simulink model "trying_HPF"  (R2024b)
settings: Solver=VariableStepAuto  StartTime=0.0  StopTime=10.0  RelTol=1e-3
libraries: simulink x4, commanapbnd3 x1
settings Model: LastModifiedBy=LENOVO

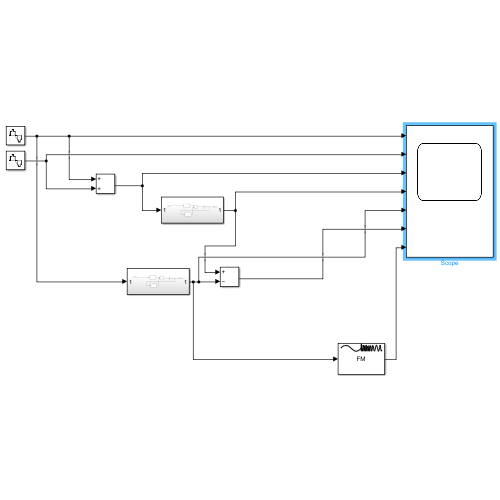
[thumbnail: Simulink's stored preview of the top-level diagram]
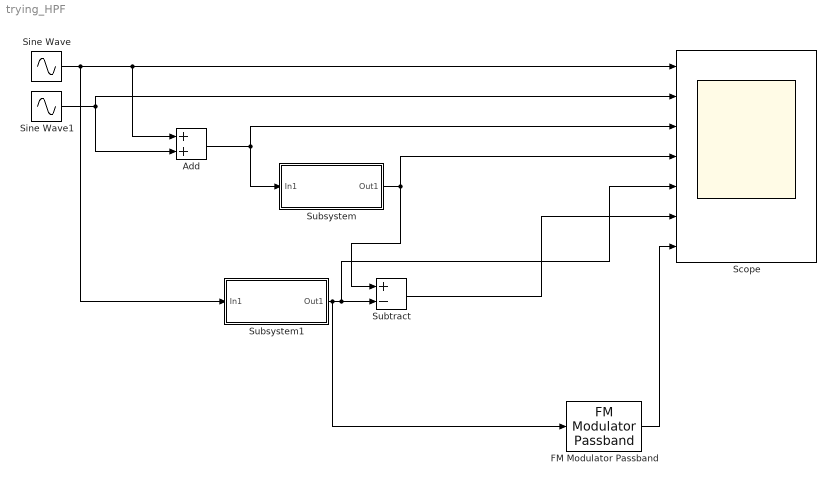
== system trying_HPF ==
  Add : Sum
  FM Modulator Passband : commanapbnd3/FM Modulator Passband  Fc=300  Ph=0  Kc=50
  Scope : Scope  NumInputPorts=7
  Sine Wave : Sin  Amplitude=2  Frequency=2*pi*0.1  SampleTime=0.001
  Sine Wave1 : Sin  Amplitude=2  Frequency=2*pi*2  SampleTime=0.001
  Subsystem : Subsystem
  Subsystem1 : Subsystem
  Subtract : Sum  Inputs=+-
  wires:
  Sine Wave/1 -> Subsystem1/1(In1), Add/1, Scope/1
  Sine Wave1/1 -> Add/2, Scope/2
  Add/1 -> Subsystem/1(In1), Scope/3
  Subsystem/1(Out1) -> Subtract/1, Scope/4
  Subsystem1/1(Out1) -> FM Modulator Passband/1, Scope/5, Subtract/2
  Subtract/1 -> Scope/6
  FM Modulator Passband/1 -> Scope/7

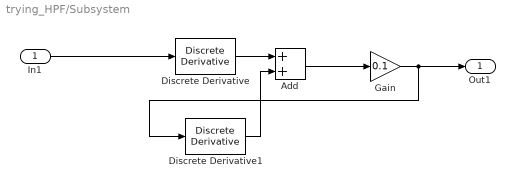
== system trying_HPF/Subsystem ==
  In1 : Inport
  Add : Sum
  Discrete Derivative : simulink/Discrete/Discrete Derivative  gainval=1.0  ICPrevScaledInput=0.0  OutMin=[]  OutMax=[]  OutDataType=fixdt(1, 16)  OutScaling=2^-10  DoSatur=off
  Discrete Derivative1 : simulink/Discrete/Discrete Derivative  gainval=1.0  ICPrevScaledInput=0.0  OutMin=[]  OutMax=[]  OutDataType=fixdt(1, 16)  OutScaling=2^-10  DoSatur=off
  Gain : Gain  Gain=0.1
  Out1 : Outport
  wires:
  Gain/1 -> Discrete Derivative1/1, Out1/1
  Add/1 -> Gain/1
  Discrete Derivative/1 -> Add/1
  In1/1 -> Discrete Derivative/1
  Discrete Derivative1/1 -> Add/2

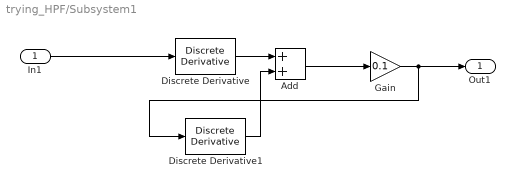
== system trying_HPF/Subsystem1 ==
  In1 : Inport
  Add : Sum
  Discrete Derivative : simulink/Discrete/Discrete Derivative  gainval=1.0  ICPrevScaledInput=0.0  OutMin=[]  OutMax=[]  OutDataType=fixdt(1, 16)  OutScaling=2^-10  DoSatur=off
  Discrete Derivative1 : simulink/Discrete/Discrete Derivative  gainval=1.0  ICPrevScaledInput=0.0  OutMin=[]  OutMax=[]  OutDataType=fixdt(1, 16)  OutScaling=2^-10  DoSatur=off
  Gain : Gain  Gain=0.1
  Out1 : Outport
  wires:
  Gain/1 -> Discrete Derivative1/1, Out1/1
  Add/1 -> Gain/1
  Discrete Derivative/1 -> Add/1
  In1/1 -> Discrete Derivative/1
  Discrete Derivative1/1 -> Add/2
